simulink model "armagentold"  (Simulink 6.2)
settings: Solver=ode45  SolverMode=SingleTasking  StartTime=0.0  StopTime=10.0  RelTol=1e-3  AbsTol=1e-6
settings Model: Creator=The MathWorks Inc.  LastModifiedBy=suarezjl  ExtModeTrigMode=oneshot  ExtModeArmWhenConnect=off  ExtModeAutoUpdateStatusClock=off
settings DataIOCC: LimitDataPoints=off  SignalLoggingName=logsOut
settings OptimizationCC: BooleanDataType=off  InlineInvariantSignals=on
settings DebuggingCC: CheckExecutionContextPreStartOutputMsg=on  CheckExecutionContextRuntimeOutputMsg=on  IntegerOverflowMsg=none
settings HardwareCC: TargetUnknown=on
settings ModelReferenceCC: UpdateModelReferenceTargets=IfOutOfDate

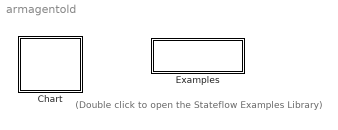
== system armagentold ==
  note: (Double click to open the
      | Stateflow Examples Library)
  Chart : Stateflow chart
  Examples : Subsystem
      settings: OpenFcn=sf('Private','sf_examples')
      mask Display: disp('Examples')

== system armagentold/Examples ==

== stateflow chart Chart ==
  state InitialArmRoutine
    Popeye\RightArm\HomingController.ComputeHomingPressures()
    Popeye\RightArm\SampleIndPressure.HW_IO_6()
    Popeye\RightArm\StateMachine.Wait(50)
  state DisableMask
    Popeye\RightArm\HomingController.Initial()
    Popeye\RightArm\SampleIndPressure.Initialize()
    Popeye\RightArm\PIDNonLinCtrl.Initial()
    Popeye\RightArm\ForwardKinematics.Initialize()
    Popeye\RightArm\InverseKinematics.Initialize()
    Popeye\RightArm\SampleIndPressure.Disable_ZMasking()
  state WriteAngles
    Popeye\RightArm\SampleIndPressure.Enable_ZMasking()
    Popeye\RightArm\SampleIndPressure.WriteHomeAngles()
  state MoveArm
    Popeye\RightArm\SampleIndPressure.HW_IO_6()
    Popeye\RightArm\PIDNonLinCtrl.PID_NonLin_6Press()
  state ComputeHomeCartesianPositions
    Popeye\RightArm\ForwardKinematics.ForwardKinematics()
    Popeye\RightArm\CopyVS.CopyCurrentVector()
    Popeye\RightArm\InverseKinematics.InverseKinematics()
  state PID_NonLinCtrlLoop
    Popeye\RightArm\PIDNonLinCtrl.PID_NonLin_12Press()
    Popeye\RightArm\SampleIndPressure.HW_IO_12()
    Popeye\RightArm\PIDNonLinCtrl.Read_CurrentPressure()
    Popeye\RightArm\ForwardKinematics.ForwardKinematics()
    Popeye\RightArm\InverseKinematics.InverseKinematics()
    Popeye\RightArm\Filter.FilterDesiredAngles()
    Popeye\RightArm\StateMachine.Wait(50)
  (default) -> DisableMask : Start
  InitialArmRoutine -> InitialArmRoutine [order 1] : Default
  DisableMask -> InitialArmRoutine : Always
  WriteAngles -> MoveArm : Always
  MoveArm -> ComputeHomeCartesianPositions : Always
  ComputeHomeCartesianPositions -> PID_NonLinCtrlLoop : Always
  PID_NonLinCtrlLoop -> PID_NonLinCtrlLoop : Always
  InitialArmRoutine -> WriteAngles [order 2] : Signal="Go to next state"
